simulink model "uavModelOrig"  (R2019a)
settings: Solver=VariableStepAuto  StartTime=0.0  StopTime=100  RelTol=1e-3
libraries: simulink x4
settings Model: Creator=tdarrah  LastModifiedBy=darrahts
settings DataIOCC: ReturnWorkspaceOutputs=off
settings DebuggingCC: ArithmeticOperatorsInVariantConditions=warning
settings SFSimCC: SimUseLocalCustomCode=off
settings RTWCC: RTWUseLocalCustomCode=off
settings CodeAppCC: StateflowObjectComments=on

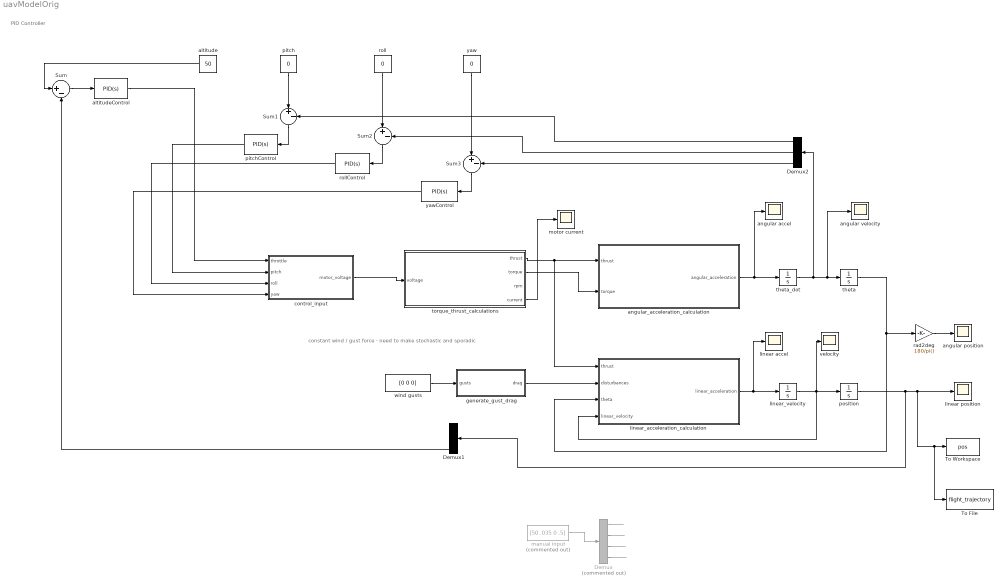
== system uavModelOrig ==
  note: constant wind / gust force
      | - need to make stochastic and sporadic
  note: PID Controller
  Demux : Demux  Commented=on
  Demux1 : Demux  Outputs=3
  Demux2 : Demux  Outputs=3
  Sum{,1..3} (4 alike) : Sum  Inputs=|+-
  To File : ToFile  Filename=flight_trajectory  MatrixName=pos  SampleTime=.1
  To Workspace : ToWorkspace  VariableName=pos  SampleTime=-1
      settings: Save2DSignal=2-D array (concatenate along first dimension)
  altitude : Constant  Value=50
  altitudeControl : simulink/Continuous/PID Controller  Controller=PID  Form=Parallel  TimeDomain=Continuous-time  SampleTime=-1  IntegratorMethod=Forward Euler  FilterMethod=Forward Euler  ControllerParametersSource=internal  P=9.031  I=1  D=10  UseFilter=on  N=100  TunerSelectOption=Transfer Function Based (PID Tuner App)  InitialConditionSource=internal  InitialConditionForIntegrator=0  InitialConditionForFilter=0  DifferentiatorICPrevScaledInput=0  ExternalReset=none  TrackingMode=off  Kt=1  LimitOutput=on  UpperSaturationLimit=100  LowerSaturationLimit=0  LinearizeAsGain=on  AntiWindupMode=clamping  Kb=1  POutMin=[]  POutMax=[]  IOutMin=[]  IOutMax=[]  DOutMin=[]  DOutMax=[]  NOutMin=[]  NOutMax=[]  SumOutMin=[]  SumOutMax=[]  SaturationOutMin=[]  SaturationOutMax=[]  PParamMin=[]  PParamMax=[]  IParamMin=[]  IParamMax=[]  DParamMin=[]  DParamMax=[]  NParamMin=[]  NParamMax=[]  KbParamMin=[]  KbParamMax=[]  KtParamMin=[]  KtParamMax=[]  KbOutMin=[]  KbOutMax=[]  KtOutMin=[]  KtOutMax=[]  IntegratorOutMin=[]  IntegratorOutMax=[]  FilterOutMin=[]  FilterOutMax=[]  SumI1OutMin=[]  SumI1OutMax=[]  SumI2OutMin=[]  SumI2OutMax=[]  SumI3OutMin=[]  SumI3OutMax=[]  SumI4OutMin=[]  SumI4OutMax=[]  SumDOutMin=[]  SumDOutMax=[]  DifferentiatorOutMin=[]  DifferentiatorOutMax=[]  FilterDiffOutCoefMin=[]  FilterDiffOutCoefMax=[]  ReciprocalOutMin=[]  ReciprocalOutMax=[]  SumDenOutMin=[]  SumDenOutMax=[]  SumNumOutMin=[]  SumNumOutMax=[]  DivideOutMin=[]  DivideOutMax=[]  IntegratorContinuousStateAttributes=''  IntegratorStateMustResolveToSignalObject=off  IntegratorRTWStateStorageClass=Auto  FilterContinuousStateAttributes=''  FilterStateMustResolveToSignalObject=off  FilterRTWStateStorageClass=Auto  ParallelPVariant=InternalParameters  IdealPVariant=Disabled  IVariant=InternalParameters  DVariant=InternalParameters  IntegratorVariant=Continuous  SatVariant=Enabled  AWVariant=ContClampingParallel  PCopyVariant=Disabled  TRVariant=Disabled  FdbkBlocksVariant=Forward  IdealPFdbkVariant=Disabled  SatFdbkVariant=Disabled  DerivativeFilterVariant=ContFilter  NVariant=InternalParameters  NCopyVariant=Disabled  FilterICVariant=InternalICsFilter  IntegratorICVariant=InternalICs  ExternalResetVariant=Disabled  TRSumVariant=Passthrough  SumFdbkVariant=Disabled  SumVariant=Sum_PID
  angular accel : Scope
  angular position : Scope
  angular velocity : Scope
  angular_acceleration_calculation : MATLAB Function  TreatAsAtomicUnit=on
  control_input : MATLAB Function  TreatAsAtomicUnit=on
  generate_gust_drag : MATLAB Function  TreatAsAtomicUnit=on
  linear accel : Scope
  linear position : Scope
  linear_acceleration_calculation : MATLAB Function  TreatAsAtomicUnit=on
  linear_velocity : Integrator
  manual input : Constant  Commented=on  Value=[50 .035 0 .5]
  motor current : Scope
  pitch : Constant  Value=0
  pitchControl : simulink/Continuous/PID Controller  Controller=PID  Form=Parallel  TimeDomain=Continuous-time  SampleTime=-1  IntegratorMethod=Forward Euler  FilterMethod=Forward Euler  ControllerParametersSource=internal  P=15  I=5  D=0  UseFilter=on  N=100  TunerSelectOption=Transfer Function Based (PID Tuner App)  InitialConditionSource=internal  InitialConditionForIntegrator=0  InitialConditionForFilter=0  DifferentiatorICPrevScaledInput=0  ExternalReset=none  TrackingMode=off  Kt=1  LimitOutput=on  UpperSaturationLimit=100  LowerSaturationLimit=0  LinearizeAsGain=on  AntiWindupMode=clamping  Kb=1  POutMin=[]  POutMax=[]  IOutMin=[]  IOutMax=[]  DOutMin=[]  DOutMax=[]  NOutMin=[]  NOutMax=[]  SumOutMin=[]  SumOutMax=[]  SaturationOutMin=[]  SaturationOutMax=[]  PParamMin=[]  PParamMax=[]  IParamMin=[]  IParamMax=[]  DParamMin=[]  DParamMax=[]  NParamMin=[]  NParamMax=[]  KbParamMin=[]  KbParamMax=[]  KtParamMin=[]  KtParamMax=[]  KbOutMin=[]  KbOutMax=[]  KtOutMin=[]  KtOutMax=[]  IntegratorOutMin=[]  IntegratorOutMax=[]  FilterOutMin=[]  FilterOutMax=[]  SumI1OutMin=[]  SumI1OutMax=[]  SumI2OutMin=[]  SumI2OutMax=[]  SumI3OutMin=[]  SumI3OutMax=[]  SumI4OutMin=[]  SumI4OutMax=[]  SumDOutMin=[]  SumDOutMax=[]  DifferentiatorOutMin=[]  DifferentiatorOutMax=[]  FilterDiffOutCoefMin=[]  FilterDiffOutCoefMax=[]  ReciprocalOutMin=[]  ReciprocalOutMax=[]  SumDenOutMin=[]  SumDenOutMax=[]  SumNumOutMin=[]  SumNumOutMax=[]  DivideOutMin=[]  DivideOutMax=[]  IntegratorContinuousStateAttributes=''  IntegratorStateMustResolveToSignalObject=off  IntegratorRTWStateStorageClass=Auto  FilterContinuousStateAttributes=''  FilterStateMustResolveToSignalObject=off  FilterRTWStateStorageClass=Auto  ParallelPVariant=InternalParameters  IdealPVariant=Disabled  IVariant=InternalParameters  DVariant=InternalParameters  IntegratorVariant=Continuous  SatVariant=Enabled  AWVariant=ContClampingParallel  PCopyVariant=Disabled  TRVariant=Disabled  FdbkBlocksVariant=Forward  IdealPFdbkVariant=Disabled  SatFdbkVariant=Disabled  DerivativeFilterVariant=ContFilter  NVariant=InternalParameters  NCopyVariant=Disabled  FilterICVariant=InternalICsFilter  IntegratorICVariant=InternalICs  ExternalResetVariant=Disabled  TRSumVariant=Passthrough  SumFdbkVariant=Disabled  SumVariant=Sum_PID
  "position " : Integrator
  rad2deg : Gain  Gain=180/pi()
  roll : Constant  Value=0
  rollControl : simulink/Continuous/PID Controller  Controller=PID  Form=Parallel  TimeDomain=Continuous-time  SampleTime=-1  IntegratorMethod=Forward Euler  FilterMethod=Forward Euler  ControllerParametersSource=internal  P=15  I=5  D=0  UseFilter=on  N=100  TunerSelectOption=Transfer Function Based (PID Tuner App)  InitialConditionSource=internal  InitialConditionForIntegrator=0  InitialConditionForFilter=0  DifferentiatorICPrevScaledInput=0  ExternalReset=none  TrackingMode=off  Kt=1  LimitOutput=on  UpperSaturationLimit=100  LowerSaturationLimit=0  LinearizeAsGain=on  AntiWindupMode=clamping  Kb=1  POutMin=[]  POutMax=[]  IOutMin=[]  IOutMax=[]  DOutMin=[]  DOutMax=[]  NOutMin=[]  NOutMax=[]  SumOutMin=[]  SumOutMax=[]  SaturationOutMin=[]  SaturationOutMax=[]  PParamMin=[]  PParamMax=[]  IParamMin=[]  IParamMax=[]  DParamMin=[]  DParamMax=[]  NParamMin=[]  NParamMax=[]  KbParamMin=[]  KbParamMax=[]  KtParamMin=[]  KtParamMax=[]  KbOutMin=[]  KbOutMax=[]  KtOutMin=[]  KtOutMax=[]  IntegratorOutMin=[]  IntegratorOutMax=[]  FilterOutMin=[]  FilterOutMax=[]  SumI1OutMin=[]  SumI1OutMax=[]  SumI2OutMin=[]  SumI2OutMax=[]  SumI3OutMin=[]  SumI3OutMax=[]  SumI4OutMin=[]  SumI4OutMax=[]  SumDOutMin=[]  SumDOutMax=[]  DifferentiatorOutMin=[]  DifferentiatorOutMax=[]  FilterDiffOutCoefMin=[]  FilterDiffOutCoefMax=[]  ReciprocalOutMin=[]  ReciprocalOutMax=[]  SumDenOutMin=[]  SumDenOutMax=[]  SumNumOutMin=[]  SumNumOutMax=[]  DivideOutMin=[]  DivideOutMax=[]  IntegratorContinuousStateAttributes=''  IntegratorStateMustResolveToSignalObject=off  IntegratorRTWStateStorageClass=Auto  FilterContinuousStateAttributes=''  FilterStateMustResolveToSignalObject=off  FilterRTWStateStorageClass=Auto  ParallelPVariant=InternalParameters  IdealPVariant=Disabled  IVariant=InternalParameters  DVariant=InternalParameters  IntegratorVariant=Continuous  SatVariant=Enabled  AWVariant=ContClampingParallel  PCopyVariant=Disabled  TRVariant=Disabled  FdbkBlocksVariant=Forward  IdealPFdbkVariant=Disabled  SatFdbkVariant=Disabled  DerivativeFilterVariant=ContFilter  NVariant=InternalParameters  NCopyVariant=Disabled  FilterICVariant=InternalICsFilter  IntegratorICVariant=InternalICs  ExternalResetVariant=Disabled  TRSumVariant=Passthrough  SumFdbkVariant=Disabled  SumVariant=Sum_PID
  theta : Integrator
  theta_dot : Integrator
  torque_thrust_calculations : MATLAB Function  TreatAsAtomicUnit=on
  velocity : Scope
  wind gusts : Constant  Value=[0 0 0]
  yaw : Constant  Value=0
  yawControl : simulink/Continuous/PID Controller  Controller=PID  Form=Parallel  TimeDomain=Continuous-time  SampleTime=-1  IntegratorMethod=Forward Euler  FilterMethod=Forward Euler  ControllerParametersSource=internal  P=15  I=5  D=0  UseFilter=on  N=100  TunerSelectOption=Transfer Function Based (PID Tuner App)  InitialConditionSource=internal  InitialConditionForIntegrator=0  InitialConditionForFilter=0  DifferentiatorICPrevScaledInput=0  ExternalReset=none  TrackingMode=off  Kt=1  LimitOutput=on  UpperSaturationLimit=100  LowerSaturationLimit=0  LinearizeAsGain=on  AntiWindupMode=clamping  Kb=1  POutMin=[]  POutMax=[]  IOutMin=[]  IOutMax=[]  DOutMin=[]  DOutMax=[]  NOutMin=[]  NOutMax=[]  SumOutMin=[]  SumOutMax=[]  SaturationOutMin=[]  SaturationOutMax=[]  PParamMin=[]  PParamMax=[]  IParamMin=[]  IParamMax=[]  DParamMin=[]  DParamMax=[]  NParamMin=[]  NParamMax=[]  KbParamMin=[]  KbParamMax=[]  KtParamMin=[]  KtParamMax=[]  KbOutMin=[]  KbOutMax=[]  KtOutMin=[]  KtOutMax=[]  IntegratorOutMin=[]  IntegratorOutMax=[]  FilterOutMin=[]  FilterOutMax=[]  SumI1OutMin=[]  SumI1OutMax=[]  SumI2OutMin=[]  SumI2OutMax=[]  SumI3OutMin=[]  SumI3OutMax=[]  SumI4OutMin=[]  SumI4OutMax=[]  SumDOutMin=[]  SumDOutMax=[]  DifferentiatorOutMin=[]  DifferentiatorOutMax=[]  FilterDiffOutCoefMin=[]  FilterDiffOutCoefMax=[]  ReciprocalOutMin=[]  ReciprocalOutMax=[]  SumDenOutMin=[]  SumDenOutMax=[]  SumNumOutMin=[]  SumNumOutMax=[]  DivideOutMin=[]  DivideOutMax=[]  IntegratorContinuousStateAttributes=''  IntegratorStateMustResolveToSignalObject=off  IntegratorRTWStateStorageClass=Auto  FilterContinuousStateAttributes=''  FilterStateMustResolveToSignalObject=off  FilterRTWStateStorageClass=Auto  ParallelPVariant=InternalParameters  IdealPVariant=Disabled  IVariant=InternalParameters  DVariant=InternalParameters  IntegratorVariant=Continuous  SatVariant=Enabled  AWVariant=ContClampingParallel  PCopyVariant=Disabled  TRVariant=Disabled  FdbkBlocksVariant=Forward  IdealPFdbkVariant=Disabled  SatFdbkVariant=Disabled  DerivativeFilterVariant=ContFilter  NVariant=InternalParameters  NCopyVariant=Disabled  FilterICVariant=InternalICsFilter  IntegratorICVariant=InternalICs  ExternalResetVariant=Disabled  TRSumVariant=Passthrough  SumFdbkVariant=Disabled  SumVariant=Sum_PID
  wires:
  torque_thrust_calculations/1(thrust) -> linear_acceleration_calculation/1(thrust), angular_acceleration_calculation/1(thrust)
  torque_thrust_calculations/2(torque) -> angular_acceleration_calculation/2(torque)
  angular_acceleration_calculation/1(angular_acceleration) -> angular accel/1, theta_dot/1
  theta_dot/1 -> Demux2/1, angular velocity/1, theta/1
  linear_acceleration_calculation/1(linear_acceleration) -> linear accel/1, linear_velocity/1
  linear_velocity/1 -> velocity/1, "position "/1, linear_acceleration_calculation/4(linear_velocity)
  generate_gust_drag/1(drag) -> linear_acceleration_calculation/2(disturbances)
  wind gusts/1 -> generate_gust_drag/1(gusts)
  control_input/1(motor_voltage) -> torque_thrust_calculations/1(voltage)
  manual input/1 -> Demux/1
  Demux/1 -> ?
  Demux/2 -> ?
  Demux/3 -> ?
  Demux/4 -> ?
  "position "/1 -> Demux1/1, To File/1, To Workspace/1, linear position/1
  rad2deg/1 -> angular position/1
  theta/1 -> rad2deg/1, linear_acceleration_calculation/3(theta)
  torque_thrust_calculations/4(current) -> motor current/1
  altitude/1 -> Sum/1
  Demux1/3 -> Sum/2
  Sum/1 -> altitudeControl/1
  Demux2/1 -> Sum1/2
  pitch/1 -> Sum1/1
  Sum1/1 -> pitchControl/1
  pitchControl/1 -> control_input/2(pitch)
  roll/1 -> Sum2/1
  Demux2/2 -> Sum2/2
  Sum2/1 -> rollControl/1
  rollControl/1 -> control_input/3(roll)
  yaw/1 -> Sum3/1
  Demux2/3 -> Sum3/2
  Sum3/1 -> yawControl/1
  yawControl/1 -> control_input/4(yaw)
  altitudeControl/1 -> control_input/1(throttle)

== matlab function uavModelOrig/angular_acceleration_calculation ==
  data: thrust input; torque input; angular_acceleration output
function angular_acceleration = calc_angular_acceleration(thrust, torque)
%
% inputs: torque vector
%         thrust vector
%
% output: rotational acceleration (of drone)
%

% moments about each axis (x,y,z) i.e. (pitch, roll, yaw)
moments = [0 0 0];

% rotational acceleration about each axis
angular_acceleration = [0 0 0];

% moments of inertia empirically derived from sample data
moments_I = [.003, .003, .007];

% pitch
% motor pair A * 1/2 rigid body length - motor pair B * rigid body length
moments(1) = (thrust(3) + thrust(4))*.237/2 - (thrust(1)+thrust(2))*.237/2;
% roll
% motor pair A * 1/2 rigid body length - motor pair B * rigid body length
moments(2) = (thrust(3) + thrust(2))*.237/2 - (thrust(1)+thrust(4))*.237/2;
%yaw
% motor pair A - motor pair B
moments(3) = (torque(4) + torque(2)) - (torque(1)  + torque(3));

for i=1:3
    angular_acceleration(i) = moments(i) / moments_I(i);
end

== matlab function uavModelOrig/torque_thrust_calculations ==
  data: voltage input; thrust output; torque output; rpm output; current output
function [thrust, torque,rpm, current] = calc_thrust_torque_current(voltage)
%
% input: voltage
%
% output: motor torque, 
%         propeller thrust 
%         battery current
%

% rpm constant
KV = 1400;
% per motor
rpm = [0 0 0 0]; 
thrust = [0 0 0 0];
torque = [0 0 0 0];
current = [0 0 0 0];

for i=1:4
    % empirically derived equation given sample data
    rpm(i) = -2.6931*voltage(i)^3 + KV*voltage(i);
    %coefficient of thrust, empirically derived
    coef_t = 2*(10^-15)*rpm(i)^3 - 4*(10^-11)*rpm(i)^2 + 3*(10^-7)*rpm(i) + .1013;
    %thrust = coef_t * density of air * velocity^2 * propeller diameter (m) ^4
    thrust(i) = coef_t*1.225*(rpm(i)/60)^2*.2^4;
    % empirically derived
    torque(i) = 4*(10^-14)*rpm(i)^3 +  8*(10^-12)*rpm(i)^2 + 3*(10^-6)*rpm(i);
    % current = rpm constant * torque
    current(i) = KV*torque(i);
end

== matlab function uavModelOrig/linear_acceleration_calculation ==
  data: thrust input; linear_acceleration output; disturbances input; theta input; linear_velocity input
function linear_acceleration = calc_linear_acceleration(thrust, disturbances, theta, linear_velocity)
%
% inputs: thrust vector (m1, m2, m3, m4)
%         disturbances vector (x,y,z)
%         theta vector (x,y,z)
%         linear velocity vector (x,y,z)
%
% output: linear acceleration vector (x,y,z)
%

m = .743; % mass of drone
g = 9.81; % acceleration due to gravity
rho = 1.225; % density of air at sea level
coef_d = 1.0; % coefficient of drag for the drone

% cross sectional areas of drone in x,y,z planes
areas = [.0197, .0197, .0512];

linear_acceleration = [0 0 0];
force = [0 0 0];
xyz_thrust = [0;0;0];
drag = [0 0 0];

% trigonometric functions for calculating pitch,roll,yaw (x,y,z) thrust 
xyz_thrust(1,1) = sin(theta(2))*cos(theta(1))*sum(thrust);
xyz_thrust(2,1) = sin(theta(1))*cos(theta(2))*sum(thrust);
xyz_thrust(3,1) = cos(theta(1))*cos(theta(2))*sum(thrust);

% angular position and magnitude on the pitch-roll (x,y) plane
angular_pos =-atan2(xyz_thrust(1), xyz_thrust(2));
angular_mag = sqrt(xyz_thrust(1)^2 + xyz_thrust(2)^2);

% if the drone is pointed upwards, x and y thrust uses + theta(3) (z)
if(xyz_thrust(3) >= 0)
    xyz_thrust(1) = angular_mag * sin(angular_pos + theta(3));
    xyz_thrust(2) = angular_mag * cos(angular_pos + theta(3));
else
    xyz_thrust(1) = angular_mag * sin(angular_pos - theta(3));
    xyz_thrust(2) = angular_mag * cos(angular_pos - theta(3));  
end

% calculate drage and force in x,y,z 
for i=1:3
    drag(i) = .5*rho*linear_velocity(i)^2* areas(i)*coef_d;
    % if the drone is going backward (w.r.t its local coordinate system)
    if (linear_velocity(i) < 0)
        force(i) = xyz_thrust(i) - disturbances(i) + drag(i);
    else
        force(i) = xyz_thrust(i) - disturbances(i) - drag(i);
    end
    % account for gravity in the z direction
    if(i == 3)
        force(i) = force(i) - m*g;
    end
end

%f=ma to calculate final acceleration
for i=1:3
    linear_acceleration(i) = force(i)/m;
end

== matlab function uavModelOrig/generate_gust_drag ==
  data: gusts input; drag output
function drag = generate_gust_drag(gusts)
%
% creates drag from wind gusts
%
% input: gusts (x,y,z)
%
% output: drag (x,y,z)
%

areas = [.0197 .0197 .0197*2*1.3];
drag = [0 0 0];
rho = 1.225;
coef_d = 1.0;

for i=1:3
    drag(i) = .5*rho*gusts(i)^2*areas(i)*coef_d;
    if(gusts(i)>0)
        drag(i) = drag(i) * -1;
    end   
end

== matlab function uavModelOrig/control_input ==
  data: throttle input; pitch input; motor_voltage output; roll input; yaw input
function motor_voltage = control_input(throttle, pitch, roll, yaw)
%
% outputs voltage per motor given control inputs
%
% inputs: throttle (double)
%         pitch (double)
%         roll (double)
%         yaw (double)
%
% output: voltage vector (m1 m2 m3 m4)
%

%battery voltage
BATT_V = 11.4;

bias = 0.0;

% pitch, roll, and yaw inputs, /2 due to drone symmetry w.r.t 4 motors
xyz_input = (pitch + roll + yaw )/2;

% difference between max throttle (100%) and current throttle
throttle_diff = 100 - throttle;

% throttle is most important, so excess is for pitch/roll/yaw
if(xyz_input > throttle_diff)
    bias = xyz_input - throttle_diff; 
end

% if the input is greater than throttle, set the bias to input-throttle
if(xyz_input > (throttle))
    if(bias < (xyz_input - throttle))
        bias = xyz_input - throttle;
    end
end

% set the bias for each motor and attitude value (pitch,roll,yaw)
bias = 2*bias/3;

%update the input commands 
if (bias ~= 0.0)
    pitch = pitch - bias;
    roll = roll - bias;
    yaw = yaw - bias;
end

motor_voltage = [(throttle - pitch/2 - roll/2 - yaw/2)*BATT_V/100
                 (throttle - pitch/2 + roll/2 + yaw/2)*BATT_V/100
                 (throttle + pitch/2 + roll/2 - yaw/2)*BATT_V/100
                 (throttle + pitch/2 - roll/2 + yaw/2)*BATT_V/100];
